simulink model "ACS"  (R2023b)
settings: Solver=FixedStepDiscrete  StartTime=0.0  StopTime=10000  FixedStep=0.01  MaxStep=10  RelTol=1e-5  AbsTol=1e-5  EnableMultiTasking=on
InitFcn:
  | initialization
undefined symbols (not defined in the file): A, AE, air_density, altitude, c_diffus, c_spec, CD, Cell_Area, CM_mm01, CM_mm02, CM_mm03, CO_mm01, CO_mm02, CO_mm03, cos50, cosines, dip_coel, dip_long, DiscIntNeverNeededParam, E_EOL, H0, inc, Inertia_tensor, K_l, k_pb, k_pe, kelly, light_speed, m_m, M_SR, magnitude, MM_Working, MT_Working, N_B, Ncell_Xn, Ncell_Xp, Ncell_Yn, Ncell_Yp, Ncell_Zn, Ncell_Zp, NX, NY, NZ, omega_BI_B0, omega_e, omega_o, omega_tx, omega_ty, omega_tz, quat_0, r, r_cm_B, r_cp_a_B, r_cp_s_B, RAAN_rt, Re, t0, TA_0, theta_g0
libraries: simulink x20, vrlib x5
(part 3 of 3)

== system ACS/Sun1/Sun Annalema/Calculating Sun position/Ecliptic Longitude (Deg) ==
  L : Inport
  g : Inport  Port=2
  Constant : Constant  Value=1.915
  Constant2 : Constant  Value=0.020
  Gain : Gain  Gain=2
  Gain1 : Gain  Gain=pi/180
  Gain2 : Gain  Gain=pi/180
  Product1 : Product  RndMeth=Zero
  Product2 : Product  RndMeth=Zero
  Sum1 : Sum  Inputs=3
  Trigonometric Function : Trigonometry
  Trigonometric Function1 : Trigonometry
  Lambda : Outport  VectorParamsAs1DForOutWhenUnconnected=off
  wires:
  Constant/1 -> Product1/1
  g/1 -> Gain/1, Gain1/1
  Constant2/1 -> Product2/2
  Gain/1 -> Gain2/1
  Trigonometric Function/1 -> Product1/2
  Trigonometric Function1/1 -> Product2/1
  Gain1/1 -> Trigonometric Function/1
  Gain2/1 -> Trigonometric Function1/1
  L/1 -> Sum1/1
  Product1/1 -> Sum1/2
  Product2/1 -> Sum1/3
  Sum1/1 -> Lambda/1

== system ACS/Sun1/Sun Annalema/Calculating Sun position/Ecuation of Time (Deg) ==
  L : Inport
  alpha : Inport  Port=2
  Gain3 : Gain  Gain=4
  Sum3 : Sum  Inputs=+-
  E : Outport  VectorParamsAs1DForOutWhenUnconnected=off
  wires:
  Sum3/1 -> Gain3/1
  L/1 -> Sum3/1
  alpha/1 -> Sum3/2
  Gain3/1 -> E/1

== system ACS/Sun1/Sun Annalema/Calculating Sun position/Mean anomaly of the Sun (Deg) ==
  n : Inport
  Constant : Constant  Value=357.528
  Constant1 : Constant  Value=0.9856003
  Product : Product  RndMeth=Zero
  Sum1 : Sum
  g : Outport  VectorParamsAs1DForOutWhenUnconnected=off
  wires:
  Constant1/1 -> Product/1
  n/1 -> Product/2
  Constant/1 -> Sum1/1
  Product/1 -> Sum1/2
  Sum1/1 -> g/1

== system ACS/Sun1/Sun Annalema/Calculating Sun position/Mean longitude of the Sun (Deg) ==
  n : Inport
  Constant : Constant  Value=280.460
  Constant1 : Constant  Value=0.9856474
  Product : Product  RndMeth=Zero
  Sum1 : Sum
  L : Outport  VectorParamsAs1DForOutWhenUnconnected=off
  wires:
  Constant/1 -> Sum1/1
  Constant1/1 -> Product/1
  n/1 -> Product/2
  Product/1 -> Sum1/2
  Sum1/1 -> L/1

== system ACS/Sun1/Sun Annalema/Calculating Sun position/Obliquity of ecliptic (Deg) ==
  n : Inport
  Constant : Constant  Value=23.439
  Constant1 : Constant  Value=0.0000004
  Product : Product  RndMeth=Zero
  Sum1 : Sum  Inputs=+-
  epsilon : Outport  VectorParamsAs1DForOutWhenUnconnected=off
  wires:
  Constant/1 -> Sum1/1
  Constant1/1 -> Product/1
  n/1 -> Product/2
  Product/1 -> Sum1/2
  Sum1/1 -> epsilon/1

== system ACS/Sun1/Sun Annalema/Calculating Sun position/Right ascension (Deg) ==
  Lambda : Inport
  epsion : Inport  Port=2
  Constant1 : Constant  Value=180/pi
  Gain1 : Gain  Gain=1/2
  Gain3 : Gain  Gain=2
  Gain4 : Gain  Gain=pi/180
  Gain5 : Gain  Gain=4
  Gain6 : Gain  Gain=pi/180
  Gain7 : Gain  Gain=1/2
  Gain8 : Gain  Gain=pi/180
  Math Function : Math  Operator=square  SignedPower=on
  Math Function1 : Math  Operator=square  SignedPower=on
  Product1 : Product  Inputs=3  RndMeth=Zero
  Product3 : Product  Inputs=3  RndMeth=Zero
  Sum1 : Sum  Inputs=+-+
  Trigonometric Function2 : Trigonometry
  Trigonometric Function3 : Trigonometry
  Trigonometric Function4 : Trigonometry  Operator=tan
  alpha : Outport  VectorParamsAs1DForOutWhenUnconnected=off
  wires:
  Lambda/1 -> Sum1/1, Gain3/1, Gain5/1
  Sum1/1 -> alpha/1
  Gain3/1 -> Gain4/1
  Gain4/1 -> Trigonometric Function2/1
  Gain5/1 -> Gain6/1
  Gain6/1 -> Trigonometric Function3/1
  epsion/1 -> Gain7/1
  Gain7/1 -> Gain8/1
  Gain8/1 -> Trigonometric Function4/1
  Trigonometric Function4/1 -> Math Function/1
  Constant1/1 -> Product3/3, Gain1/1
  Math Function/1 -> Product3/2, Math Function1/1
  Trigonometric Function2/1 -> Product3/1
  Trigonometric Function3/1 -> Product1/1
  Math Function1/1 -> Product1/2
  Gain1/1 -> Product1/3
  Product1/1 -> Sum1/3
  Product3/1 -> Sum1/2

== system ACS/Earth/Simple model of Earth's Magnetic Field1/Simple model of Earth's Magnetic Field1/Simple Magnetc Field/Earths magnetic field in Inertial frame1 ==
  R_ECEF : Inport
  dd_ECEF : Inport  Port=2
  TS : Inport  Port=3
  Divide : Product  Inputs=*/
  Divide1 : Product  Inputs=***
  Divide5 : Product  Inputs=**
  Divide6 : Product  Inputs=*/
  Dot Product : DotProduct  OutDataTypeStr=Inherit: Inherit via internal rule
  If : If  IfExpression=(u1 > eps | u1 < -eps)
  If Action Subsystem : Subsystem  TreatAsAtomicUnit=on
  If Action Subsystem1 : Subsystem  TreatAsAtomicUnit=on
  Math Function : Math  Operator=pow  SignedPower=on
  Merge : Merge
  Sum : Sum  Inputs=+-
  magnetic_field8 : ToWorkspace  VariableName=Rdotm  SampleTime=-1
  sat distance from Earth's CM3 : Constant  Value=r
  sat distance from Earth's CM : Constant  Value=r
  sat distance from Earth's CM1 : Constant  Value=3
  sat distance from Earth's CM3 : Constant  Value=3
  B_ECEF : Outport  VectorParamsAs1DForOutWhenUnconnected=off
  wires:
  Sum/1 -> Divide5/2
  dd_ECEF/1 -> Sum/2, Dot Product/2
  Divide6/1 -> Divide1/1, Dot Product/1
  sat distance from Earth's CM3/1 -> Divide6/2
  R_ECEF/1 -> Divide6/1
  TS/1 -> Divide/1
  sat distance from Earth's CM/1 -> Math Function/1
  sat distance from Earth's CM1/1 -> Math Function/2
  Math Function/1 -> Divide/2
  Divide/1 -> Divide5/1
  Divide5/1 -> B_ECEF/1
  sat distance from Earth's CM3/1 -> Divide1/2
  Divide1/1 -> Sum/1
  If/1 -> If Action Subsystem/Action
  If Action Subsystem/1(Out1) -> Merge/1
  Merge/1 -> magnetic_field8/1, Divide1/3
  If Action Subsystem1/1(Out1) -> Merge/2
  If/2 -> If Action Subsystem1/Action
  Dot Product/1 -> If/1, If Action Subsystem/1(In1)

== system ACS/Perturbations/perturbation_Torque1/Solar Torque and Force Calculation/Force_toque1/force on X+ ==
  P : Inport
  A_xp : Inport  Port=2
  theta_xp : Inport  Port=3
  C_S : Inport  Port=4
  C_D : Inport  Port=5
  S_ES_B : Inport  Port=6
  Constant : Constant
  Divide{1..2,4..5} (4 alike) : Product
  Divide3 : Product  Inputs=***
  Gain : Gain  Gain=1/3
  Gain1 : Gain  Gain=2
  Gain2 : Gain  Gain=-1
  Normal : Constant  Value=[1 0 0]
  Saturation : Saturate  UpperLimit=1  LowerLimit=0
  Sum : Sum  Inputs=+-
  Sum1 : Sum
  Sum2 : Sum  Inputs=2
  Trigonometric Function1 : Trigonometry  Operator=cos
  F_s_xp : Outport  VectorParamsAs1DForOutWhenUnconnected=off
  wires:
  Saturation/1 -> Divide3/1, Divide1/2
  Divide5/1 -> F_s_xp/1
  Sum2/1 -> Divide5/2
  Divide4/1 -> Sum2/1
  S_ES_B/1 -> Divide4/1
  Divide2/1 -> Sum2/2
  Normal/1 -> Divide2/2
  Gain1/1 -> Divide2/1
  Sum1/1 -> Gain1/1
  Gain/1 -> Sum1/2
  Divide1/1 -> Sum1/1
  C_D/1 -> Gain/1
  Sum/1 -> Divide4/2
  C_S/1 -> Divide1/1, Sum/2
  Constant/1 -> Sum/1
  theta_xp/1 -> Trigonometric Function1/1
  Trigonometric Function1/1 -> Saturation/1
  P/1 -> Divide3/2
  A_xp/1 -> Divide3/3
  Divide3/1 -> Gain2/1
  Gain2/1 -> Divide5/1

== system ACS/Perturbations/perturbation_Torque1/Solar Torque and Force Calculation/Force_toque1/force on X- ==
  P : Inport
  A_xm : Inport  Port=2
  theta_xm : Inport  Port=3
  C_S : Inport  Port=4
  C_D : Inport  Port=5
  S_ES_B : Inport  Port=6
  Constant : Constant
  Divide{1..2,4..5} (4 alike) : Product
  Divide3 : Product  Inputs=***
  Gain : Gain  Gain=1/3
  Gain1 : Gain  Gain=2
  Gain2 : Gain  Gain=-1
  Normal : Constant  Value=[-1 0 0]
  Saturation : Saturate  UpperLimit=1  LowerLimit=0
  Sum : Sum  Inputs=+-
  Sum1 : Sum
  Sum2 : Sum  Inputs=2
  Trigonometric Function1 : Trigonometry  Operator=cos
  F_s_xm : Outport  VectorParamsAs1DForOutWhenUnconnected=off
  wires:
  Gain2/1 -> Divide5/1
  Divide3/1 -> Gain2/1
  A_xm/1 -> Divide3/3
  P/1 -> Divide3/2
  Trigonometric Function1/1 -> Saturation/1
  theta_xm/1 -> Trigonometric Function1/1
  Constant/1 -> Sum/1
  C_S/1 -> Sum/2, Divide1/1
  Sum/1 -> Divide4/2
  C_D/1 -> Gain/1
  Divide1/1 -> Sum1/1
  Gain/1 -> Sum1/2
  Sum1/1 -> Gain1/1
  Gain1/1 -> Divide2/1
  Normal/1 -> Divide2/2
  Divide2/1 -> Sum2/2
  S_ES_B/1 -> Divide4/1
  Divide4/1 -> Sum2/1
  Sum2/1 -> Divide5/2
  Divide5/1 -> F_s_xm/1
  Saturation/1 -> Divide1/2, Divide3/1

== system ACS/Perturbations/perturbation_Torque1/Solar Torque and Force Calculation/Force_toque1/force on Y+ ==
  P : Inport
  A_yp : Inport  Port=2
  theta_yp : Inport  Port=3
  C_S : Inport  Port=4
  C_D : Inport  Port=5
  S_ES_B : Inport  Port=6
  Constant : Constant
  Divide{1..2,4..5} (4 alike) : Product
  Divide3 : Product  Inputs=***
  Gain : Gain  Gain=1/3
  Gain1 : Gain  Gain=2
  Gain2 : Gain  Gain=-1
  Normal : Constant  Value=[0 1 0]
  Saturation : Saturate  UpperLimit=1  LowerLimit=0
  Sum : Sum  Inputs=+-
  Sum1 : Sum
  Sum2 : Sum  Inputs=2
  Trigonometric Function1 : Trigonometry  Operator=cos
  F_s_yp : Outport  VectorParamsAs1DForOutWhenUnconnected=off
  wires:
  Saturation/1 -> Divide3/1, Divide1/2
  Divide5/1 -> F_s_yp/1
  Sum2/1 -> Divide5/2
  Divide4/1 -> Sum2/1
  S_ES_B/1 -> Divide4/1
  Divide2/1 -> Sum2/2
  Normal/1 -> Divide2/2
  Gain1/1 -> Divide2/1
  Sum1/1 -> Gain1/1
  Gain/1 -> Sum1/2
  Divide1/1 -> Sum1/1
  C_D/1 -> Gain/1
  Sum/1 -> Divide4/2
  C_S/1 -> Divide1/1, Sum/2
  Constant/1 -> Sum/1
  theta_yp/1 -> Trigonometric Function1/1
  Trigonometric Function1/1 -> Saturation/1
  P/1 -> Divide3/2
  A_yp/1 -> Divide3/3
  Divide3/1 -> Gain2/1
  Gain2/1 -> Divide5/1

== system ACS/Perturbations/perturbation_Torque1/Solar Torque and Force Calculation/Force_toque1/force on Y- ==
  P : Inport
  A_ym : Inport  Port=2
  theta_ym : Inport  Port=3
  C_S : Inport  Port=4
  C_D : Inport  Port=5
  S_ES_B : Inport  Port=6
  Constant : Constant
  Divide{1..2,4..5} (4 alike) : Product
  Divide3 : Product  Inputs=***
  Gain : Gain  Gain=1/3
  Gain1 : Gain  Gain=2
  Gain2 : Gain  Gain=-1
  Normal : Constant  Value=[0 -1 0]
  Saturation : Saturate  UpperLimit=1  LowerLimit=0
  Sum : Sum  Inputs=+-
  Sum1 : Sum
  Sum2 : Sum  Inputs=2
  Trigonometric Function1 : Trigonometry  Operator=cos
  F_s_ym : Outport  VectorParamsAs1DForOutWhenUnconnected=off
  wires:
  Saturation/1 -> Divide3/1, Divide1/2
  Divide5/1 -> F_s_ym/1
  Sum2/1 -> Divide5/2
  Divide4/1 -> Sum2/1
  S_ES_B/1 -> Divide4/1
  Divide2/1 -> Sum2/2
  Normal/1 -> Divide2/2
  Gain1/1 -> Divide2/1
  Sum1/1 -> Gain1/1
  Gain/1 -> Sum1/2
  Divide1/1 -> Sum1/1
  C_D/1 -> Gain/1
  Sum/1 -> Divide4/2
  C_S/1 -> Divide1/1, Sum/2
  Constant/1 -> Sum/1
  theta_ym/1 -> Trigonometric Function1/1
  Trigonometric Function1/1 -> Saturation/1
  P/1 -> Divide3/2
  A_ym/1 -> Divide3/3
  Divide3/1 -> Gain2/1
  Gain2/1 -> Divide5/1

== system ACS/Perturbations/perturbation_Torque1/Solar Torque and Force Calculation/Force_toque1/force on Z+ ==
  P : Inport
  A_zp : Inport  Port=2
  theta_zp : Inport  Port=3
  C_S : Inport  Port=4
  C_D : Inport  Port=5
  S_ES_B : Inport  Port=6
  Constant : Constant
  Divide{1..2,4..5} (4 alike) : Product
  Divide3 : Product  Inputs=***
  Gain : Gain  Gain=1/3
  Gain1 : Gain  Gain=2
  Gain2 : Gain  Gain=-1
  Normal : Constant  Value=[0 0 1]
  Saturation : Saturate  UpperLimit=1  LowerLimit=0
  Sum : Sum  Inputs=+-
  Sum1 : Sum
  Sum2 : Sum  Inputs=2
  Trigonometric Function1 : Trigonometry  Operator=cos
  F_s_zp : Outport  VectorParamsAs1DForOutWhenUnconnected=off
  wires:
  Gain2/1 -> Divide5/1
  Divide3/1 -> Gain2/1
  A_zp/1 -> Divide3/3
  P/1 -> Divide3/2
  Trigonometric Function1/1 -> Saturation/1
  theta_zp/1 -> Trigonometric Function1/1
  Constant/1 -> Sum/1
  C_S/1 -> Sum/2, Divide1/1
  Sum/1 -> Divide4/2
  C_D/1 -> Gain/1
  Divide1/1 -> Sum1/1
  Gain/1 -> Sum1/2
  Sum1/1 -> Gain1/1
  Gain1/1 -> Divide2/1
  Normal/1 -> Divide2/2
  Divide2/1 -> Sum2/2
  S_ES_B/1 -> Divide4/1
  Divide4/1 -> Sum2/1
  Sum2/1 -> Divide5/2
  Divide5/1 -> F_s_zp/1
  Saturation/1 -> Divide1/2, Divide3/1

== system ACS/Perturbations/perturbation_Torque1/Solar Torque and Force Calculation/Force_toque1/force on Z- ==
  P : Inport
  A_zm : Inport  Port=2
  theta_zm : Inport  Port=3
  C_S : Inport  Port=4
  C_D : Inport  Port=5
  S_ES_B : Inport  Port=6
  Constant : Constant
  Divide{1..2,4..5} (4 alike) : Product
  Divide3 : Product  Inputs=***
  Gain : Gain  Gain=1/3
  Gain1 : Gain  Gain=2
  Gain2 : Gain  Gain=-1
  Normal : Constant  Value=[0 0 -1]
  Saturation : Saturate  UpperLimit=1  LowerLimit=0
  Sum : Sum  Inputs=+-
  Sum1 : Sum
  Sum2 : Sum  Inputs=2
  Trigonometric Function1 : Trigonometry  Operator=cos
  F_s_zm : Outport  VectorParamsAs1DForOutWhenUnconnected=off
  wires:
  Saturation/1 -> Divide3/1, Divide1/2
  Divide5/1 -> F_s_zm/1
  Sum2/1 -> Divide5/2
  Divide4/1 -> Sum2/1
  S_ES_B/1 -> Divide4/1
  Divide2/1 -> Sum2/2
  Normal/1 -> Divide2/2
  Gain1/1 -> Divide2/1
  Sum1/1 -> Gain1/1
  Gain/1 -> Sum1/2
  Divide1/1 -> Sum1/1
  C_D/1 -> Gain/1
  Sum/1 -> Divide4/2
  C_S/1 -> Divide1/1, Sum/2
  Constant/1 -> Sum/1
  theta_zm/1 -> Trigonometric Function1/1
  Trigonometric Function1/1 -> Saturation/1
  P/1 -> Divide3/2
  A_zm/1 -> Divide3/3
  Divide3/1 -> Gain2/1
  Gain2/1 -> Divide5/1

== system ACS/Satellite/OBC/Nominal Attitude Control/Control/Control law ==
  B_dot : Inport
  B : Inport  Port=2
  omega : Inport  Port=3
  k_pb : Inport  Port=4
  k_pe : Inport  Port=5
  Cross Product : vrlib/Utilities/Cross Product
  Gain3 : Gain  Gain=-1
  Math Function : Math  Operator=10^u  SignedPower=on
  Product : Product  Inputs=3
  Sum : Sum  Inputs=2
  M : Outport  VectorParamsAs1DForOutWhenUnconnected=off
  wires:
  B/1 -> Cross Product/2
  Gain3/1 -> M/1
  Sum/1 -> Product/1
  B_dot/1 -> Sum/1
  Cross Product/1 -> Sum/2
  Product/1 -> Gain3/1
  Math Function/1 -> Product/3
  k_pb/1 -> Product/2
  k_pe/1 -> Math Function/1
  omega/1 -> Cross Product/1

== system ACS/Satellite/OBC/Nominal Attitude Control/Control/If Fail Recalculate ==
  M : Inport
  B_b_T : Inport  Port=2
  Working : Inport  Port=3
  1 Fail : Subsystem
  2 Fails : Subsystem
  Compare To Constant1 : simulink/Logic and Bit Operations/Compare To Constant  relop===  const=1  OutDataTypeStr=uint8  ZeroCross=off
  Compare To Constant2 : simulink/Logic and Bit Operations/Compare To Constant  relop===  const=2  OutDataTypeStr=uint8  ZeroCross=off
  Compare To Constant3 : simulink/Logic and Bit Operations/Compare To Constant  relop===  const=3  OutDataTypeStr=uint8  ZeroCross=off
  Noone Fails1 : Subsystem
  Sum of Elements1 : Sum  Inputs=+
  Sum of Elements2 : Sum  Inputs=+
  Sum of Elements3 : Sum  Inputs=+
  Sum1 : Sum  Inputs=3
  I_A : Outport  VectorParamsAs1DForOutWhenUnconnected=off
  wires:
  Compare To Constant1/1 -> 2 Fails/Enable
  2 Fails/1(M_xyz) -> Sum1/3
  Sum of Elements3/1 -> Compare To Constant1/1
  Sum of Elements2/1 -> Compare To Constant3/1
  Sum of Elements1/1 -> Compare To Constant2/1
  M/1 -> 2 Fails/2(M), 1 Fail/2(M), Noone Fails1/1(M)
  Compare To Constant2/1 -> 1 Fail/Enable
  Compare To Constant3/1 -> Noone Fails1/Enable
  1 Fail/1(M_xyz) -> Sum1/2
  Noone Fails1/1(M_xyz) -> Sum1/1
  B_b_T/1 -> 1 Fail/3(B)
  Working/1 -> Sum of Elements2/1, 2 Fails/1(Fail), Sum of Elements3/1, 1 Fail/1(Fail), Sum of Elements1/1
  Sum1/1 -> I_A/1

== system ACS/Satellite/OBC/Nominal Attitude Control/Control/Limitation ==
  M : Inport
  "m_m " : Inport  Port=2
  Demux : Demux  Outputs=3
  Limitation : Subsystem
  Limitation1 : Subsystem
  Limitation2 : Subsystem
  Mux : Mux  Inputs=3
  MT : Outport  VectorParamsAs1DForOutWhenUnconnected=off
  wires:
  Mux/1 -> MT/1
  Limitation1/1(MT) -> Mux/2
  Limitation2/1(MT) -> Mux/3
  Limitation/1(MT) -> Mux/1
  "m_m "/1 -> Limitation2/2("m_m "), Limitation1/2("m_m "), Limitation/2("m_m ")
  M/1 -> Demux/1
  Demux/1 -> Limitation/1(M)
  Demux/2 -> Limitation1/1(M)
  Demux/3 -> Limitation2/1(M)

== system ACS/Satellite/OBC/Nominal Attitude Control/Control/Magnetic field calculation ==
  B_b_T1 : Inport
  Derivative : Subsystem
  Media : Subsystem
  B_dot : Outport  VectorParamsAs1DForOutWhenUnconnected=off
  B_med : Outport  Port=2  VectorParamsAs1DForOutWhenUnconnected=off
  wires:
  B_b_T1/1 -> Derivative/1(In1), Media/1(B_b_T_1s)
  Media/1(B_b_T_1s_m) -> B_med/1
  Derivative/1(B_dot) -> B_dot/1

== system ACS/Satellite/OBC/Nominal Attitude Control/Control/discretization ==
  PD : Inport
  m_m : Inport  Port=2
  Abs : Abs  SaturateOnIntegerOverflow=off
  Compare To Constant : simulink/Logic and Bit Operations/Compare To Constant  relop=>=  const=0.2  OutDataTypeStr=uint8  ZeroCross=off
  Data Type Conversion : DataTypeConversion  SaturateOnIntegerOverflow=off  RndMeth=Floor
  Gain1 : Gain  Gain=10
  Gain3 : Gain  Gain=0.1
  Gain4 : Gain  Gain=0.5
  Gain5 : Gain  Gain=1/(0.25)
  Memory : Memory  InheritSampleTime=on
  Product : Product  RndMeth=Zero
  Product1 : Product  Inputs=*/  RndMeth=Zero
  Rounding Function : Rounding  Operator=round
  Sum : Sum  Inputs=+-
  Sum1 : Sum  Inputs=2
  MT : Outport  VectorParamsAs1DForOutWhenUnconnected=off
  wires:
  Rounding Function/1 -> Gain3/1
  Gain1/1 -> Rounding Function/1
  Sum/1 -> Memory/1
  Sum1/1 -> Gain1/1, Sum/1
  Gain3/1 -> Abs/1, Product/1
  Compare To Constant/1 -> Data Type Conversion/1
  Data Type Conversion/1 -> Product/2
  Abs/1 -> Compare To Constant/1
  PD/1 -> Gain5/1
  Product/1 -> MT/1, Sum/2
  Memory/1 -> Sum1/1
  Gain4/1 -> Sum1/2
  Gain5/1 -> Product1/1
  Product1/1 -> Gain4/1
  m_m/1 -> Product1/2

== system ACS/Satellite/OBC/Nominal Attitude Control/Sensor/Average ==
  B_b_T : Inport
  MM_working : Inport  Port=2
  Bus Selector : BusSelector  OutputSignals=B_MM1,B_MM2,B_MM3
  Demux : Demux  Outputs=3
  Product : Product
  Product1 : Product
  Product2 : Product
  Product3 : Product  Inputs=*/
  Sum : Sum  Inputs=3
  Sum of Elements : Sum  Inputs=+
  B_b_T_1s : Outport  VectorParamsAs1DForOutWhenUnconnected=off
  wires:
  MM_working/1 -> Demux/1, Sum of Elements/1
  Demux/1 -> Product/2  "MM1_working"
  Demux/2 -> Product1/2  "MM2_working"
  Demux/3 -> Product2/2  "MM3_Working"
  Product/1 -> Sum/1
  Product1/1 -> Sum/2
  Product2/1 -> Sum/3
  Sum/1 -> Product3/1
  Product3/1 -> B_b_T_1s/1
  Sum of Elements/1 -> Product3/2
  B_b_T/1 -> Bus Selector/1
  Bus Selector/1 -> Product/1  "<B_MM1>"
  Bus Selector/2 -> Product1/1  "<B_MM2>"
  Bus Selector/3 -> Product2/1  "<B_MM3>"

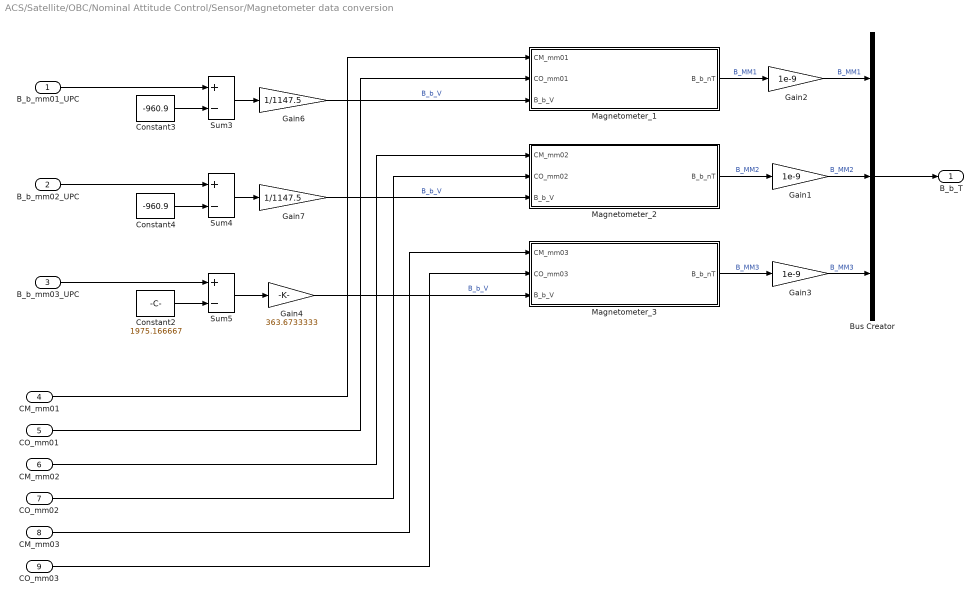
== system ACS/Satellite/OBC/Nominal Attitude Control/Sensor/Magnetometer data conversion  ==
  B_b_mm01_UPC : Inport
  B_b_mm02_UPC : Inport  Port=2
  B_b_mm03_UPC : Inport  Port=3
  CM_mm01 : Inport  Port=4
  CO_mm01 : Inport  Port=5
  CM_mm02 : Inport  Port=6
  CO_mm02 : Inport  Port=7
  CM_mm03 : Inport  Port=8
  CO_mm03 : Inport  Port=9
  Bus Creator : BusCreator  Inputs=3
  Constant2 : Constant  Value=1975.166667  OutDataTypeStr=single
  Constant3 : Constant  Value=-960.9  OutDataTypeStr=single
  Constant4 : Constant  Value=-960.9  OutDataTypeStr=single
  Gain1 : Gain  Gain=1e-9
  Gain2 : Gain  Gain=1e-9
  Gain3 : Gain  Gain=1e-9
  Gain4 : Gain  Gain=363.6733333
  Gain6 : Gain  Gain=1/1147.5
  Gain7 : Gain  Gain=1/1147.5
  Magnetometer_1 : Subsystem
  Magnetometer_2 : Subsystem
  Magnetometer_3 : Subsystem
  Sum3 : Sum  Inputs=+-
  Sum4 : Sum  Inputs=+-
  Sum5 : Sum  Inputs=+-
  B_b_T : Outport  VectorParamsAs1DForOutWhenUnconnected=off
  wires:
  Magnetometer_1/1(B_b_nT) -> Gain2/1  "B_MM1"
  Magnetometer_2/1(B_b_nT) -> Gain1/1  "B_MM2"
  B_b_mm02_UPC/1 -> Sum4/1
  Bus Creator/1 -> B_b_T/1
  Gain2/1 -> Bus Creator/1  "B_MM1"
  Gain1/1 -> Bus Creator/2  "B_MM2"
  Gain3/1 -> Bus Creator/3  "B_MM3"
  B_b_mm03_UPC/1 -> Sum5/1
  Magnetometer_3/1(B_b_nT) -> Gain3/1  "B_MM3"
  B_b_mm01_UPC/1 -> Sum3/1
  Sum3/1 -> Gain6/1
  Sum4/1 -> Gain7/1
  Sum5/1 -> Gain4/1
  Gain6/1 -> Magnetometer_1/3(B_b_V)  "B_b_V"
  Gain7/1 -> Magnetometer_2/3(B_b_V)  "B_b_V"
  Gain4/1 -> Magnetometer_3/3(B_b_V)  "B_b_V"
  Constant3/1 -> Sum3/2
  Constant4/1 -> Sum4/2
  Constant2/1 -> Sum5/2
  CM_mm01/1 -> Magnetometer_1/1(CM_mm01)
  CO_mm01/1 -> Magnetometer_1/2(CO_mm01)
  CM_mm02/1 -> Magnetometer_2/1(CM_mm02)
  CO_mm02/1 -> Magnetometer_2/2(CO_mm02)
  CM_mm03/1 -> Magnetometer_3/1(CM_mm03)
  CO_mm03/1 -> Magnetometer_3/2(CO_mm03)

== system ACS/Satellite/OBC/Nominal Attitude Control/Sensor/Memory ==
  B_b_T : Inport
  Mux : Mux  Inputs=5
  Terminator : Terminator
  Unit Delay{,1..4} (5 alike) : UnitDelay  SampleTime=-1  HasFrameUpgradeWarning=on
  B_b_T_1s : Outport  VectorParamsAs1DForOutWhenUnconnected=off
  wires:
  Unit Delay4/1 -> Terminator/1, Mux/5
  Mux/1 -> B_b_T_1s/1
  Unit Delay3/1 -> Unit Delay4/1, Mux/4
  Unit Delay2/1 -> Unit Delay3/1, Mux/3
  Unit Delay1/1 -> Unit Delay2/1, Mux/2
  Unit Delay/1 -> Unit Delay1/1, Mux/1
  B_b_T/1 -> Unit Delay/1

== system ACS/Earth/Simple model of Earth's Magnetic Field1/Simple model of Earth's Magnetic Field1/Simple Magnetc Field/Earths magnetic field in Inertial frame1/If Action Subsystem ==
  In1 : Inport
  Action Port : ActionPort  ActionPortLabel=if((u1 > eps | u1 < -eps) )
  Out1 : Outport  VectorParamsAs1DForOutWhenUnconnected=off
  wires:
  In1/1 -> Out1/1

== system ACS/Earth/Simple model of Earth's Magnetic Field1/Simple model of Earth's Magnetic Field1/Simple Magnetc Field/Earths magnetic field in Inertial frame1/If Action Subsystem1 ==
  Action Port : ActionPort  ActionPortLabel=else
  sat distance from Earth's CM3 : Constant  Value=0
  Out1 : Outport  VectorParamsAs1DForOutWhenUnconnected=off
  wires:
  sat distance from Earth's CM3/1 -> Out1/1

== system ACS/Satellite/OBC/Nominal Attitude Control/Control/If Fail Recalculate/1 Fail ==
  Fail : Inport
  M : Inport  Port=2
  B : Inport  Port=3
  Enable : EnablePort
  B_tot : Subsystem
  Cross Product : vrlib/Utilities/Cross Product
  Fails X : Subsystem
  Fails Y : Subsystem
  Fails Z : Subsystem
  Logical Operator : Logic  Operator=NOT  AllPortsSameDT=off  OutDataTypeStr=boolean
  Selector : Selector  InputPortWidth=3  IndexOptions=Index vector (dialog)  Indices=[1]  OutputSizes=1
  Selector1 : Selector  InputPortWidth=3  IndexOptions=Index vector (dialog)  Indices=[2]  OutputSizes=1
  Selector2 : Selector  InputPortWidth=3  IndexOptions=Index vector (dialog)  Indices=[3]  OutputSizes=1
  Sum : Sum  Inputs=3
  M_xyz : Outport  VectorParamsAs1DForOutWhenUnconnected=off
  wires:
  Sum/1 -> M_xyz/1
  M/1 -> Cross Product/1
  B/1 -> Cross Product/2, B_tot/1(B)
  B_tot/1(B_tot) -> Fails X/1(B_tot), Fails Y/1(B_tot), Fails Z/1(B_tot)
  B_tot/2(b) -> Fails Y/2(b), Fails Z/2(b), Fails X/2(b)
  Cross Product/1 -> Fails X/3(T_Nm), Fails Y/3(T_Nm), Fails Z/3(T_Nm)
  Fails X/1(M_yz) -> Sum/1
  Fails Y/1(M_yz) -> Sum/2
  Fails Z/1(M_xy) -> Sum/3
  Selector/1 -> Fails X/Enable
  Selector1/1 -> Fails Y/Enable
  Selector2/1 -> Fails Z/Enable
  Fail/1 -> Logical Operator/1
  Logical Operator/1 -> Selector/1, Selector1/1, Selector2/1

== system ACS/Satellite/OBC/Nominal Attitude Control/Control/If Fail Recalculate/2 Fails ==
  Fail : Inport
  M : Inport  Port=2
  Enable : EnablePort
  Demux1 : Demux  Outputs=3
  Demux3 : Demux  Outputs=3
  Mux : Mux  Inputs=3
  Product : Product  RndMeth=Zero
  Product1 : Product  RndMeth=Zero
  Product2 : Product  RndMeth=Zero
  M_xyz : Outport  VectorParamsAs1DForOutWhenUnconnected=off
  wires:
  Mux/1 -> M_xyz/1
  M/1 -> Demux3/1
  Product2/1 -> Mux/3
  Product1/1 -> Mux/2
  Product/1 -> Mux/1
  Demux3/1 -> Product/1
  Demux3/2 -> Product1/1
  Demux3/3 -> Product2/1
  Demux1/3 -> Product2/2
  Demux1/2 -> Product1/2
  Fail/1 -> Demux1/1
  Demux1/1 -> Product/2

== system ACS/Satellite/OBC/Nominal Attitude Control/Control/If Fail Recalculate/Noone Fails1 ==
  M : Inport
  Enable : EnablePort
  M_xyz : Outport  VectorParamsAs1DForOutWhenUnconnected=off
  wires:
  M/1 -> M_xyz/1

== system ACS/Satellite/OBC/Nominal Attitude Control/Control/Limitation/Limitation ==
  M : Inport
  "m_m " : Inport  Port=2
  Gain : Gain  Gain=-1
  If : If  NumInputs=2  IfExpression=u1 > u2  ElseIfExpressions=u1 < -u2
  If Action Subsystem : Subsystem  TreatAsAtomicUnit=on
  If Action Subsystem1 : Subsystem  TreatAsAtomicUnit=on
  If Action Subsystem2 : Subsystem  TreatAsAtomicUnit=on
  Merge : Merge  Inputs=3
  MT : Outport  VectorParamsAs1DForOutWhenUnconnected=off
  wires:
  "m_m "/1 -> If Action Subsystem/1(In1), Gain/1, If/2
  If/1 -> If Action Subsystem/Action
  M/1 -> If Action Subsystem2/1(In1), If/1
  If Action Subsystem/1(Out1) -> Merge/1
  If Action Subsystem1/1(Out1) -> Merge/2
  Merge/1 -> MT/1
  If/2 -> If Action Subsystem1/Action
  If/3 -> If Action Subsystem2/Action
  If Action Subsystem2/1(Out1) -> Merge/3
  Gain/1 -> If Action Subsystem1/1(In1)

== system ACS/Satellite/OBC/Nominal Attitude Control/Control/Limitation/Limitation1 ==
  M : Inport
  "m_m " : Inport  Port=2
  Gain : Gain  Gain=-1
  If : If  NumInputs=2  IfExpression=u1 > u2  ElseIfExpressions=u1 < -u2
  If Action Subsystem : Subsystem  TreatAsAtomicUnit=on
  If Action Subsystem1 : Subsystem  TreatAsAtomicUnit=on
  If Action Subsystem2 : Subsystem  TreatAsAtomicUnit=on
  Merge : Merge  Inputs=3
  MT : Outport  VectorParamsAs1DForOutWhenUnconnected=off
  wires:
  Gain/1 -> If Action Subsystem1/1(In1)
  If Action Subsystem2/1(Out1) -> Merge/3
  If/3 -> If Action Subsystem2/Action
  If/2 -> If Action Subsystem1/Action
  Merge/1 -> MT/1
  If Action Subsystem1/1(Out1) -> Merge/2
  If Action Subsystem/1(Out1) -> Merge/1
  M/1 -> If/1, If Action Subsystem2/1(In1)
  If/1 -> If Action Subsystem/Action
  "m_m "/1 -> If/2, Gain/1, If Action Subsystem/1(In1)

== system ACS/Satellite/OBC/Nominal Attitude Control/Control/Limitation/Limitation2 ==
  M : Inport
  "m_m " : Inport  Port=2
  Gain : Gain  Gain=-1
  If : If  NumInputs=2  IfExpression=u1 > u2  ElseIfExpressions=u1 < -u2
  If Action Subsystem : Subsystem  TreatAsAtomicUnit=on
  If Action Subsystem1 : Subsystem  TreatAsAtomicUnit=on
  If Action Subsystem2 : Subsystem  TreatAsAtomicUnit=on
  Merge : Merge  Inputs=3
  MT : Outport  VectorParamsAs1DForOutWhenUnconnected=off
  wires:
  "m_m "/1 -> If Action Subsystem/1(In1), Gain/1, If/2
  If/1 -> If Action Subsystem/Action
  M/1 -> If Action Subsystem2/1(In1), If/1
  If Action Subsystem/1(Out1) -> Merge/1
  If Action Subsystem1/1(Out1) -> Merge/2
  Merge/1 -> MT/1
  If/2 -> If Action Subsystem1/Action
  If/3 -> If Action Subsystem2/Action
  If Action Subsystem2/1(Out1) -> Merge/3
  Gain/1 -> If Action Subsystem1/1(In1)

== system ACS/Satellite/OBC/Nominal Attitude Control/Control/Magnetic field calculation/Derivative ==
  In1 : Inport
  Gain : Gain  Gain=-1
  Gain1 : Gain  Gain=-1
  Gain2 : Gain  Gain=-1
  Mux : Mux  Inputs=3
  Polyfit : Subsystem
  Polyfit1 : Subsystem
  Polyfit2 : Subsystem
  Selector3 : Selector  InputPortWidth=15  IndexOptions=Index vector (dialog)  Indices=[1:3:13]  OutputSizes=1
  Selector4 : Selector  InputPortWidth=15  IndexOptions=Index vector (dialog)  Indices=[2:3:14]  OutputSizes=1
  Selector5 : Selector  InputPortWidth=15  IndexOptions=Index vector (dialog)  Indices=[3:3:15]  OutputSizes=1
  B_dot : Outport  VectorParamsAs1DForOutWhenUnconnected=off
  wires:
  In1/1 -> Selector3/1, Selector4/1, Selector5/1
  Mux/1 -> B_dot/1
  Gain/1 -> Mux/1
  Gain1/1 -> Mux/2
  Gain2/1 -> Mux/3
  Selector3/1 -> Polyfit/1(U)
  Selector4/1 -> Polyfit1/1(U)
  Selector5/1 -> Polyfit2/1(U)
  Polyfit/1(A) -> Gain/1
  Polyfit1/1(A) -> Gain1/1
  Polyfit2/1(A) -> Gain2/1

== system ACS/Satellite/OBC/Nominal Attitude Control/Control/Magnetic field calculation/Media ==
  B_b_T_1s : Inport
  Demux : Demux  Outputs=5
  Gain : Gain  Gain=1/5
  Sum1 : Sum  Inputs=5
  B_b_T_1s_m : Outport  VectorParamsAs1DForOutWhenUnconnected=off
  wires:
  Sum1/1 -> Gain/1
  Gain/1 -> B_b_T_1s_m/1
  B_b_T_1s/1 -> Demux/1
  Demux/1 -> Sum1/1
  Demux/2 -> Sum1/2
  Demux/3 -> Sum1/3
  Demux/4 -> Sum1/4
  Demux/5 -> Sum1/5

== system ACS/Satellite/OBC/Nominal Attitude Control/Sensor/Magnetometer data conversion /Magnetometer_1 ==
  CM_mm01 : Inport
  CO_mm01 : Inport  Port=2
  B_b_V : Inport  Port=3
  Product : Product  Multiplication=Matrix(*)  RndMeth=Zero
  Sum : Sum  Inputs=-+
  B_b_nT : Outport  VectorParamsAs1DForOutWhenUnconnected=off
  wires:
  B_b_V/1 -> Sum/2
  Sum/1 -> Product/2
  Product/1 -> B_b_nT/1
  CO_mm01/1 -> Sum/1
  CM_mm01/1 -> Product/1

== system ACS/Satellite/OBC/Nominal Attitude Control/Sensor/Magnetometer data conversion /Magnetometer_2 ==
  CM_mm02 : Inport
  CO_mm02 : Inport  Port=2
  B_b_V : Inport  Port=3
  Product : Product  Multiplication=Matrix(*)  RndMeth=Zero
  Sum : Sum  Inputs=-+
  B_b_nT : Outport  VectorParamsAs1DForOutWhenUnconnected=off
  wires:
  B_b_V/1 -> Sum/2
  Sum/1 -> Product/2
  Product/1 -> B_b_nT/1
  CM_mm02/1 -> Product/1
  CO_mm02/1 -> Sum/1

== system ACS/Satellite/OBC/Nominal Attitude Control/Sensor/Magnetometer data conversion /Magnetometer_3 ==
  CM_mm03 : Inport
  CO_mm03 : Inport  Port=2
  B_b_V : Inport  Port=3
  Product : Product  Multiplication=Matrix(*)  RndMeth=Zero
  Sum : Sum  Inputs=-+
  B_b_nT : Outport  VectorParamsAs1DForOutWhenUnconnected=off
  wires:
  B_b_V/1 -> Sum/2
  Sum/1 -> Product/2
  Product/1 -> B_b_nT/1
  CO_mm03/1 -> Sum/1
  CM_mm03/1 -> Product/1

== system ACS/Satellite/OBC/Nominal Attitude Control/Control/If Fail Recalculate/1 Fail/B_tot ==
  B : Inport
  Add : Sum  Inputs=+++
  Compare To Zero : simulink/Logic and Bit Operations/Compare To Zero  relop===  OutDataTypeStr=uint8  ZeroCross=off
  Demux : Demux  Outputs=3
  Math Function : Math  Operator=magnitude^2  SignedPower=on
  Math Function1 : Math  Operator=magnitude^2  SignedPower=on
  Math Function2 : Math  Operator=magnitude^2  SignedPower=on
  Math Function3 : Math  Operator=sqrt  SignedPower=on
  Product4 : Product  Inputs=*/  RndMeth=Zero
  Sum : Sum  Inputs=|++
  B_tot : Outport  VectorParamsAs1DForOutWhenUnconnected=off
  b : Outport  Port=2  VectorParamsAs1DForOutWhenUnconnected=off
  wires:
  Demux/1 -> Math Function/1
  Demux/2 -> Math Function1/1
  Demux/3 -> Math Function2/1
  Math Function/1 -> Add/1
  Math Function1/1 -> Add/2
  Math Function2/1 -> Add/3
  Add/1 -> Math Function3/1
  B/1 -> Demux/1, Product4/1
  Math Function3/1 -> Sum/1, Compare To Zero/1
  Sum/1 -> B_tot/1, Product4/2
  Compare To Zero/1 -> Sum/2
  Product4/1 -> b/1

== system ACS/Satellite/OBC/Nominal Attitude Control/Control/If Fail Recalculate/1 Fail/Fails X ==
  B_tot : Inport
  b : Inport  Port=2
  T_Nm : Inport  Port=3
  Enable : EnablePort
  Constant : Constant  Value=0  OutDataTypeStr=single
  Matrix x-fails : Subsystem
  Mux : Mux  Inputs=2
  Product1 : Product  Multiplication=Matrix(*)  RndMeth=Zero
  Product3 : Product  Inputs=/*  RndMeth=Zero
  M_yz : Outport  VectorParamsAs1DForOutWhenUnconnected=off
  wires:
  Matrix x-fails/1(M2) -> Product1/1
  T_Nm/1 -> Product1/2
  Product1/1 -> Product3/2
  Product3/1 -> Mux/2
  Mux/1 -> M_yz/1
  B_tot/1 -> Product3/1
  b/1 -> Matrix x-fails/1(b)
  Constant/1 -> Mux/1

== system ACS/Satellite/OBC/Nominal Attitude Control/Control/If Fail Recalculate/1 Fail/Fails Y ==
  B_tot : Inport
  b : Inport  Port=2
  T_Nm : Inport  Port=3
  Enable : EnablePort
  Constant : Constant  Value=0  OutDataTypeStr=single
  Demux : Demux  Outputs=2
  Matrix y-fails : Subsystem
  Mux : Mux  Inputs=3
  Product1 : Product  Multiplication=Matrix(*)  RndMeth=Zero
  Product3 : Product  Inputs=/*  RndMeth=Zero
  M_yz : Outport  VectorParamsAs1DForOutWhenUnconnected=off
  wires:
  b/1 -> Matrix y-fails/1(b)
  B_tot/1 -> Product3/1
  Mux/1 -> M_yz/1
  Product1/1 -> Product3/2
  T_Nm/1 -> Product1/2
  Matrix y-fails/1(M2) -> Product1/1
  Product3/1 -> Demux/1
  Demux/1 -> Mux/1
  Demux/2 -> Mux/3
  Constant/1 -> Mux/2

== system ACS/Satellite/OBC/Nominal Attitude Control/Control/If Fail Recalculate/1 Fail/Fails Z ==
  B_tot : Inport
  b : Inport  Port=2
  T_Nm : Inport  Port=3
  Enable : EnablePort
  Constant : Constant  Value=0  OutDataTypeStr=single
  Matrix z-fails : Subsystem
  Mux : Mux  Inputs=2
  Product1 : Product  Multiplication=Matrix(*)  RndMeth=Zero
  Product3 : Product  Inputs=/*  RndMeth=Zero
  M_xy : Outport  VectorParamsAs1DForOutWhenUnconnected=off
  wires:
  Matrix z-fails/1(M2) -> Product1/1
  T_Nm/1 -> Product1/2
  Product1/1 -> Product3/2
  Mux/1 -> M_xy/1
  B_tot/1 -> Product3/1
  b/1 -> Matrix z-fails/1(b)
  Product3/1 -> Mux/1
  Constant/1 -> Mux/2

== system ACS/Satellite/OBC/Nominal Attitude Control/Control/Limitation/Limitation/If Action Subsystem ==
  In1 : Inport
  Action Port : ActionPort  ActionPortLabel=if(u1 > u2)
  Out1 : Outport  VectorParamsAs1DForOutWhenUnconnected=off
  wires:
  In1/1 -> Out1/1

== system ACS/Satellite/OBC/Nominal Attitude Control/Control/Limitation/Limitation/If Action Subsystem1 ==
  In1 : Inport
  Action Port : ActionPort  ActionPortLabel=elseif(u1 < -u2)
  Out1 : Outport  VectorParamsAs1DForOutWhenUnconnected=off
  wires:
  In1/1 -> Out1/1

== system ACS/Satellite/OBC/Nominal Attitude Control/Control/Limitation/Limitation/If Action Subsystem2 ==
  In1 : Inport
  Action Port : ActionPort  ActionPortLabel=else
  Out1 : Outport  VectorParamsAs1DForOutWhenUnconnected=off
  wires:
  In1/1 -> Out1/1

== system ACS/Satellite/OBC/Nominal Attitude Control/Control/Limitation/Limitation1/If Action Subsystem ==
  In1 : Inport
  Action Port : ActionPort  ActionPortLabel=if(u1 > u2)
  Out1 : Outport  VectorParamsAs1DForOutWhenUnconnected=off
  wires:
  In1/1 -> Out1/1

== system ACS/Satellite/OBC/Nominal Attitude Control/Control/Limitation/Limitation1/If Action Subsystem1 ==
  In1 : Inport
  Action Port : ActionPort  ActionPortLabel=elseif(u1 < -u2)
  Out1 : Outport  VectorParamsAs1DForOutWhenUnconnected=off
  wires:
  In1/1 -> Out1/1

== system ACS/Satellite/OBC/Nominal Attitude Control/Control/Limitation/Limitation1/If Action Subsystem2 ==
  In1 : Inport
  Action Port : ActionPort  ActionPortLabel=else
  Out1 : Outport  VectorParamsAs1DForOutWhenUnconnected=off
  wires:
  In1/1 -> Out1/1

== system ACS/Satellite/OBC/Nominal Attitude Control/Control/Limitation/Limitation2/If Action Subsystem ==
  In1 : Inport
  Action Port : ActionPort  ActionPortLabel=if(u1 > u2)
  Out1 : Outport  VectorParamsAs1DForOutWhenUnconnected=off
  wires:
  In1/1 -> Out1/1

== system ACS/Satellite/OBC/Nominal Attitude Control/Control/Limitation/Limitation2/If Action Subsystem1 ==
  In1 : Inport
  Action Port : ActionPort  ActionPortLabel=elseif(u1 < -u2)
  Out1 : Outport  VectorParamsAs1DForOutWhenUnconnected=off
  wires:
  In1/1 -> Out1/1

== system ACS/Satellite/OBC/Nominal Attitude Control/Control/Limitation/Limitation2/If Action Subsystem2 ==
  In1 : Inport
  Action Port : ActionPort  ActionPortLabel=else
  Out1 : Outport  VectorParamsAs1DForOutWhenUnconnected=off
  wires:
  In1/1 -> Out1/1

== system ACS/Satellite/OBC/Nominal Attitude Control/Control/Magnetic field calculation/Derivative/Polyfit ==
  U : Inport
  N : Constant  Value=5  OutDataTypeStr=single
  NSx2 : Product  Inputs=*/
  NSxx : Product
  NSxy : Product
  Sum{,1..2,5} (4 alike) : Sum  Inputs=+
  Sum3 : Sum  Inputs=+-
  Sum4 : Sum  Inputs=+-
  SxSx : Product
  "SxSy " : Product
  Sxx : Product
  Sxy : Product
  time : Constant  Value=[1:5]/5  OutDataTypeStr=single
  A : Outport  VectorParamsAs1DForOutWhenUnconnected=off
  wires:
  U/1 -> Sxy/2, Sum/1
  time/1 -> Sxx/2, Sxx/1, Sxy/1, Sum1/1
  N/1 -> NSxx/1, NSxy/1
  Sxy/1 -> Sum2/1
  NSxy/1 -> Sum3/1
  Sum1/1 -> SxSx/2, SxSx/1, "SxSy "/1
  Sum/1 -> "SxSy "/2
  "SxSy "/1 -> Sum3/2
  NSx2/1 -> A/1
  Sxx/1 -> Sum5/1
  NSxx/1 -> Sum4/1
  SxSx/1 -> Sum4/2
  Sum3/1 -> NSx2/1
  Sum4/1 -> NSx2/2
  Sum2/1 -> NSxy/2
  Sum5/1 -> NSxx/2

== system ACS/Satellite/OBC/Nominal Attitude Control/Control/Magnetic field calculation/Derivative/Polyfit1 ==
  U : Inport
  N : Constant  Value=5  OutDataTypeStr=single
  NSx2 : Product  Inputs=*/
  NSxx : Product
  NSxy : Product
  Sum{,1..2,5} (4 alike) : Sum  Inputs=+
  Sum3 : Sum  Inputs=+-
  Sum4 : Sum  Inputs=+-
  SxSx : Product
  "SxSy " : Product
  Sxx : Product
  Sxy : Product
  time : Constant  Value=[1:5]/5  OutDataTypeStr=single
  A : Outport  VectorParamsAs1DForOutWhenUnconnected=off
  wires:
  Sum5/1 -> NSxx/2
  Sum2/1 -> NSxy/2
  Sum4/1 -> NSx2/2
  Sum3/1 -> NSx2/1
  SxSx/1 -> Sum4/2
  NSxx/1 -> Sum4/1
  Sxx/1 -> Sum5/1
  NSx2/1 -> A/1
  "SxSy "/1 -> Sum3/2
  Sum/1 -> "SxSy "/2
  Sum1/1 -> "SxSy "/1, SxSx/1, SxSx/2
  NSxy/1 -> Sum3/1
  Sxy/1 -> Sum2/1
  N/1 -> NSxy/1, NSxx/1
  time/1 -> Sum1/1, Sxy/1, Sxx/1, Sxx/2
  U/1 -> Sum/1, Sxy/2

== system ACS/Satellite/OBC/Nominal Attitude Control/Control/Magnetic field calculation/Derivative/Polyfit2 ==
  U : Inport
  N : Constant  Value=5  OutDataTypeStr=single
  NSx2 : Product  Inputs=*/
  NSxx : Product
  NSxy : Product
  Sum{,1..2,5} (4 alike) : Sum  Inputs=+
  Sum3 : Sum  Inputs=+-
  Sum4 : Sum  Inputs=+-
  SxSx : Product
  "SxSy " : Product
  Sxx : Product
  Sxy : Product
  time : Constant  Value=[1:5]/5  OutDataTypeStr=single
  A : Outport  VectorParamsAs1DForOutWhenUnconnected=off
  wires:
  U/1 -> Sxy/2, Sum/1
  time/1 -> Sxx/2, Sxx/1, Sxy/1, Sum1/1
  N/1 -> NSxx/1, NSxy/1
  Sxy/1 -> Sum2/1
  NSxy/1 -> Sum3/1
  Sum1/1 -> SxSx/2, SxSx/1, "SxSy "/1
  Sum/1 -> "SxSy "/2
  "SxSy "/1 -> Sum3/2
  NSx2/1 -> A/1
  Sxx/1 -> Sum5/1
  NSxx/1 -> Sum4/1
  SxSx/1 -> Sum4/2
  Sum3/1 -> NSx2/1
  Sum4/1 -> NSx2/2
  Sum2/1 -> NSxy/2
  Sum5/1 -> NSxx/2

== system ACS/Satellite/OBC/Nominal Attitude Control/Control/If Fail Recalculate/1 Fail/Fails X/Matrix x-fails ==
  b : Inport
  Fcn10 : Fcn  Expr=(1-u(2)^2)/(u(1)+Delta*(u(1)==0))
  Fcn5 : Fcn  Expr=(u(3))
  Fcn6 : Fcn  Expr=-(u(2))
  Fcn7 : Fcn  Expr=(u(2)*u(3))/(u(1)+Delta*(u(1)==0))
  Fcn8 : Fcn  Expr=-(u(2)*u(3))/(u(1)+Delta*(u(1)==0))
  Fcn9 : Fcn  Expr=-(1-u(3)^2)/(u(1)+Delta*(u(1)==0))
  Mux : Mux  Inputs=6
  Reshape : Reshape  OutputDimensionality=Customize  OutputDimensions=[2,3]
  M2 : Outport  VectorParamsAs1DForOutWhenUnconnected=off
  wires:
  Fcn5/1 -> Mux/1
  b/1 -> Fcn5/1, Fcn6/1, Fcn10/1, Fcn9/1, Fcn8/1, Fcn7/1
  Reshape/1 -> M2/1
  Mux/1 -> Reshape/1
  Fcn6/1 -> Mux/2
  Fcn7/1 -> Mux/3
  Fcn8/1 -> Mux/6
  Fcn10/1 -> Mux/4
  Fcn9/1 -> Mux/5

== system ACS/Satellite/OBC/Nominal Attitude Control/Control/If Fail Recalculate/1 Fail/Fails Y/Matrix y-fails ==
  b : Inport
  Fcn1 : Fcn  Expr=(u(1)*u(3))/(u(2)+Delta*(u(2)==0))
  Fcn2 : Fcn  Expr=(1-u(3)^2)/(u(2)+Delta*(u(2)==0))
  Fcn3 : Fcn  Expr=(u(1))
  Fcn5 : Fcn  Expr=-(u(3))
  Fcn8 : Fcn  Expr=-(u(1)*u(3))/(u(2)+Delta*(u(2)==0))
  Fcn9 : Fcn  Expr=-(1-u(1)^2)/(u(2)+Delta*(u(2)==0))
  Mux : Mux  Inputs=6
  Reshape : Reshape  OutputDimensionality=Customize  OutputDimensions=[2,3]
  M2 : Outport  VectorParamsAs1DForOutWhenUnconnected=off
  wires:
  Fcn2/1 -> Mux/5
  Fcn3/1 -> Mux/4
  Fcn1/1 -> Mux/6
  Fcn5/1 -> Mux/3
  Mux/1 -> Reshape/1
  Reshape/1 -> M2/1
  b/1 -> Fcn1/1, Fcn2/1, Fcn3/1, Fcn5/1, Fcn8/1, Fcn9/1
  Fcn9/1 -> Mux/2
  Fcn8/1 -> Mux/1

== system ACS/Satellite/OBC/Nominal Attitude Control/Control/If Fail Recalculate/1 Fail/Fails Z/Matrix z-fails ==
  b : Inport
  Fcn1 : Fcn  Expr=-(u(2)*u(1))/(u(3)+Delta*(u(3)==0))
  Fcn10 : Fcn  Expr=(1-u(1)^2)/(u(3)+Delta*(u(3)==0))
  Fcn2 : Fcn  Expr=-(u(1))
  Fcn3 : Fcn  Expr=-(1-u(2)^2)/(u(3)+Delta*(u(3)==0))
  Fcn6 : Fcn  Expr=(u(2))
  Fcn7 : Fcn  Expr=(u(2)*u(1))/(u(3)+Delta*(u(3)==0))
  Mux : Mux  Inputs=6
  Reshape : Reshape  OutputDimensionality=Customize  OutputDimensions=[2,3]
  M2 : Outport  VectorParamsAs1DForOutWhenUnconnected=off
  wires:
  b/1 -> Fcn7/1, Fcn10/1, Fcn6/1, Fcn2/1, Fcn1/1, Fcn3/1
  Reshape/1 -> M2/1
  Mux/1 -> Reshape/1
  Fcn3/1 -> Mux/3
  Fcn2/1 -> Mux/6
  Fcn1/1 -> Mux/4
  Fcn6/1 -> Mux/5
  Fcn7/1 -> Mux/1
  Fcn10/1 -> Mux/2
